simulink model "regulator_ver2"  (Simulink 8.4)
settings: Solver=ode5  StartTime=0.0  StopTime=500  FixedStep=0.05  RelTol=1e-3
values from neighbouring files (symbols this model uses):
  a = 31    [charakterystyka_pompa.m]    (also in charakterystyka_pompa_sterownik.m; dane14listopad.mat; danePompa.mat; pomiary.m)
  b = 40    [charakterystyki_zawory_reczne.m]    (also in daneZawory_cz2.mat; pomiary.m; rhs.m)
  c = p(1)    [cel.m]    (also in charakterystyki_zawory_reczne.m = 10; daneZawory_cz2.mat = 10; identyfikacja_parametrow.m = 10; identyfikacja_zawor2.m = 10)
  C1 = q/sqrt(H1pp)    [linearyzacja_analitycznie.m]    (also in wskaznikZawor1.m = parametry(1))
  C2 = q/sqrt(H2pp)    [linearyzacja_analitycznie.m]    (also in wskaznikZawor2.m = parametry(1))
  C3 = q/sqrt(H3pp)    [linearyzacja_analitycznie.m]    (also in wskaznikZawor3.m = parametry(1))
  H2max = 40    [charakterystyki_zawory_reczne.m]    (also in daneZawory_cz2.mat; pomiary.m)
  R = 40    [charakterystyki_zawory_reczne.m]    (also in daneZawory_cz2.mat; nastawyLQ.m; pomiary.m; rhs.m)
  w = 5    [charakterystyka_pompa.m]    (also in charakterystyka_pompa_sterownik.m; dane14listopad.mat; danePompa.mat; pomiary.m)
settings Model: Creator=Michal  LastModifiedBy=Michal
settings DataIOCC: SignalLoggingSaveFormat=Dataset
settings OptimizationCC: ExpressionDepthLimit=128
settings DebuggingCC: ArtificialAlgebraicLoopMsg=none  FcnCallInpInsideContextMsg=EnableAllAsError  StateNameClashWarn=none
settings GRTTargetCC: CombineOutputUpdateFcns=on  GRTInterface=off
settings ConfigComp: Description=PLC Coder Custom Configuration Component  PLC_TargetIDE=pcworx60  PLC_GenerateReport=off

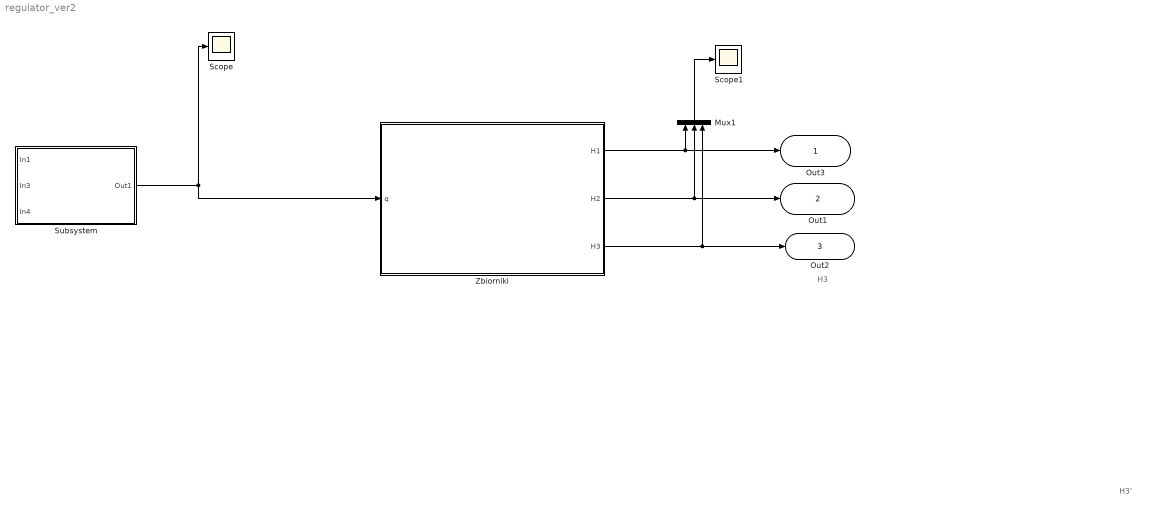
== system regulator_ver2 ==
  note: H3
  note: H3'
  Mux1 : Mux  Inputs=3
  Scope : Scope
      settings: TimeRange=500  SaveName=q_lqr
  Scope1 : Scope
      settings: TimeRange=500  YMin=-300000  YMax=50000  SaveName=H_lqr
  Subsystem : Subsystem  TreatAsAtomicUnit=on
      settings: MinAlgLoopOccurrences=on
  Zbiorniki : Subsystem
  Out3 : Outport
  Out1 : Outport  Port=2
  Out2 : Outport  Port=3
  wires:
  Zbiorniki/3(H3) -> Out2/1, Mux1/3
  Zbiorniki/1(H1) -> Mux1/1, Out3/1
  Zbiorniki/2(H2) -> Mux1/2, Out1/1
  Mux1/1 -> Scope1/1
  Subsystem/1(Out1) -> Zbiorniki/1(q), Scope/1

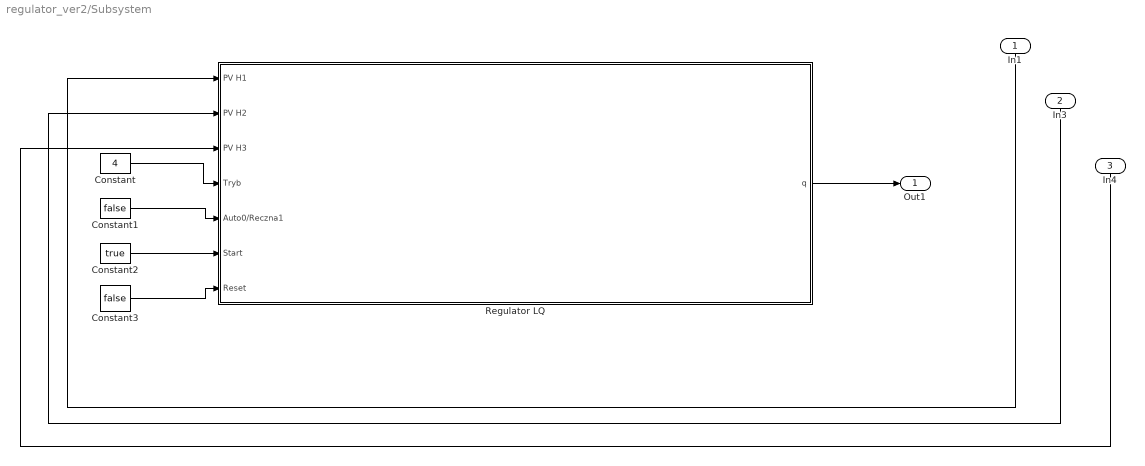
== system regulator_ver2/Subsystem ==
  In1 : Inport  OutDataTypeStr=single
  In3 : Inport  Port=2  OutDataTypeStr=single
  In4 : Inport  Port=3  OutDataTypeStr=single
  Constant : Constant  Value=4  OutDataTypeStr=uint16
  Constant1 : Constant  Value=false  OutMin=0  OutMax=1  OutDataTypeStr=boolean
  Constant2 : Constant  Value=true  OutMin=0  OutMax=1  OutDataTypeStr=boolean
  Constant3 : Constant  Value=false  OutMin=0  OutMax=1  OutDataTypeStr=boolean
  Regulator LQ : Subsystem  TreatAsAtomicUnit=on
      settings: MinAlgLoopOccurrences=on
  Out1 : Outport
  wires:
  In1/1 -> Regulator LQ/1(PV H1)
  In4/1 -> Regulator LQ/3(PV H3)
  In3/1 -> Regulator LQ/2(PV H2)
  Constant/1 -> Regulator LQ/4(Tryb)
  Constant1/1 -> Regulator LQ/5(Auto0/Reczna1)
  Regulator LQ/1(q) -> Out1/1
  Constant2/1 -> Regulator LQ/6(Start)
  Constant3/1 -> Regulator LQ/7(Reset)

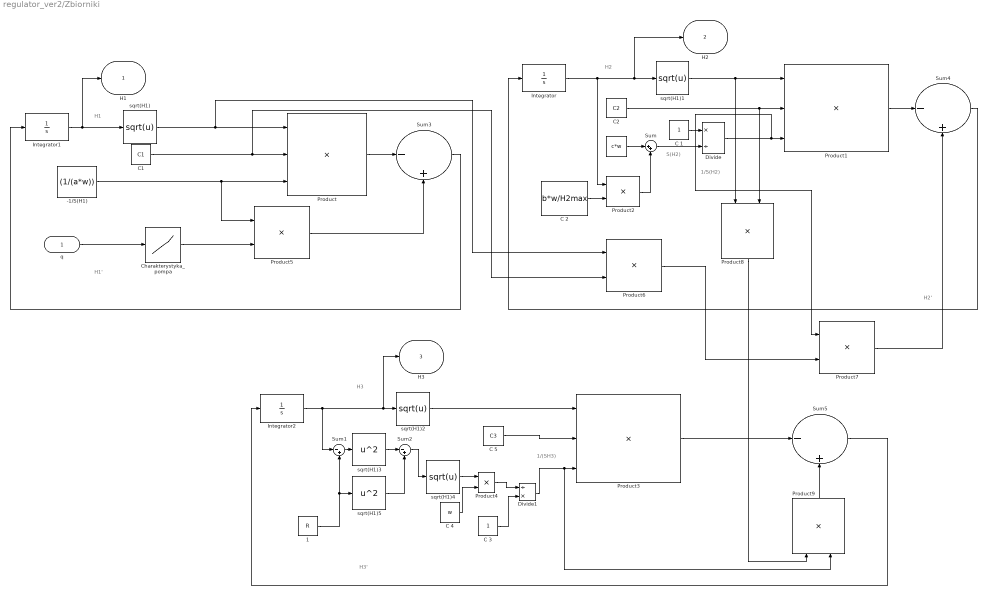
== system regulator_ver2/Zbiorniki ==
  note: H1
  note: 1/S(H2)
  note: S(H2)
  note: H2'
  note: H2
  note: 1/(SH3)
  note: H3
  note: H1'
  note: H3'
  q : Inport
  " " : Constant  Value=c*w
  " 1" : Constant  Value=R
  -1/S(H1) : Constant  Value=(1/(a*w))
  C 1 : Constant
  C 2 : Constant  Value=b*w/H2max
  C 3 : Constant
  C 4 : Constant  Value=w
  C 5 : Constant  Value=C3
  "C1 " : Constant  Value=C1
  "C2 " : Constant  Value=C2
  Charakterystyka_pompa : Lookup_n-D  NumberOfTableDimensions=1  BreakpointsForDimension1="[0.300000000000000\t0.305000000000000\t0.310000000000000\t0.315000000000000\t0.320000000000000\t0.325000000000000\t0.330000000000000\t0.335000000000000\t0.340000000000000\t0.345000000000000\t0.350000000000000\t0.355000000000000\t0.360000000000000\t0.365000000000000\t0.370000000000000\t0.375000000000000\t0.380000000000000\t0.385000000000000\t0.390000000000000\t0.395000000000000\t0.400000000000000\t0.405000000000000\t0.410000000000000\t0.415000000000000\t0.420000000000000\t0.425000000000000\t0.430000000000000\t0.435000000000000\t0.440000000000000\t0.445000000000000\t0.450000000000000\t0.455000000000000\t0.460000000000000\t0.465000000000000\t0.470000000000000\t0.475000000000000\t0.480000000000000\t0.485000000000000\t0.490000000000000\t0.495000000000000\t0.500000000000000\t0.505000000000000\t0.510000000000000\t0.515000000000000\t0.520000000000000\t0.525000000000000\t0.530000000000000\t0.535000000000000\t0.540000000000000\t0.545000000000000\t0.550000000000000\t0.555000000000000\t0.560000000000000\t0.565000000000000\t0.570000000000000\t0.575000000000000\t0.580000000000000\t0.585000000000000\t0.590000000000000\t0.595000000000000\t0.600000000000000\t0.605000000000000\t0.610000000000000\t0.615000000000000\t0.620000000000000\t0.625000000000000\t0.630000000000000\t0.635000000000000\t0.640000000000000\t0.645000000000000\t0.650000000000000\t0.655000000000000\t0.660000000000000\t0.665000000000000\t0.670000000000000\t0.675000000000000\t0.680000000000000\t0.685000000000000\t0.690000000000000\t0.695000000000000\t0.700000000000000\t0.705000000000000\t0.710000000000000\t0.715000000000000\t0.720000000000000\t0.725000000000000\t0.730000000000000\t0.735000000000000\t0.740000000000000\t0.745000000000000\t0.750000000000000\t0.755000000000000\t0.760000000000000\t0.765000000000000\t0.770000000000000\t0.775000000000000\t0.780000000000000\t0.785000000000000\t0.790000000000000\t0.795000000000000\t0.800000000000000\t0.805000000000000\t0.810000000000000\t0.815000000000000\t0.820000000000000\t0.825000000000000\t0.830000000000000\t0.835000000000000\t0.840000000000000\t0.845000000000000\t0.850000000000000\t0.855000000000000\t0.860000000000000\t0.865000000000000\t0.870000000000000\t0.875000000000000\t0.880000000000000\t0.885000000000000\t0.890000000000000\t0.895000000000000\t0.900000000000000\t0.905000000000000\t0.910000000000000\t0.915000000000000\t0.920000000000000\t0.925000000000000\t0.930000000000000\t0.935000000000000\t0.940000000000000\t0.945000000000000\t0.950000000000000\t0.955000000000000\t0.960000000000000\t0.965000000000000\t0.970000000000000\t0.975000000000000\t0.980000000000000\t0.985000000000000\t0.990000000000000\t0.995000000000000\t1]"  Table="[10.4471978396270\t11.7296031510510\t13.0028115267443\t14.2669102745871\t15.5219867024602\t16.7681281182441\t18.0054218298192\t19.2339551450661\t20.4538153718654\t21.6650898180975\t22.8678657916430\t24.0622306003825\t25.2482715521964\t26.4260759549652\t27.5957311165696\t28.7573243448901\t29.9109429478071\t31.0566742332013\t32.1946055089531\t33.3248240829430\t34.4474172630516\t35.5624723571595\t36.6700766731472\t37.7703175188951\t38.8632822022838\t39.9490580311939\t41.0277323135059\t42.0993923571003\t43.1641254698577\t44.2220189596585\t45.2731601343833\t46.3176363019127\t47.3555347701271\t48.3869428469072\t49.4119478401333\t50.4306370576861\t51.4430978074461\t52.4494173972938\t53.4496831351098\t54.4439823287746\t55.4324022861686\t56.4150303151725\t57.3919537236668\t58.3632598195320\t59.3290359106486\t60.2893693048972\t61.2443473101582\t62.1940572343123\t63.1385863852399\t64.0780220708216\t65.0124515989380\t65.9419622774695\t66.8666414142967\t67.7865763173000\t68.7018542943601\t69.6125626533575\t70.5187887021727\t71.4206197486861\t72.3181431007785\t73.2114460663303\t74.1006159532220\t74.9857400693341\t75.8669057225472\t76.7442002207418\t77.6177108717985\t78.4875249835977\t79.3537298640200\t80.2164128209460\t81.0756611622562\t81.9315621958310\t82.7842032295510\t83.6336715712968\t84.4800545289489\t85.3234394103878\t86.1639135234941\t87.0015641761482\t87.8364786762308\t88.6687443316223\t89.4984484502032\t90.3256783398542\t91.1505213084557\t91.9730646638883\t92.7933957140324\t93.6116017667686\t94.4277701299776\t95.2419881115397\t96.0543430193355\t96.8649221612455\t97.6738128451504\t98.4811023789305\t99.2868780704665\t100.091227227639\t100.894237158328\t101.695995170415\t102.496588571779\t103.296104670302\t104.094630773865\t104.892254190346\t105.689062227628\t106.485142193590\t107.280581396114\t108.075467143079\t108.869886742366\t109.663927501857\t110.457676729430\t111.251221732967\t112.044649820349\t112.838048299455\t113.631504478167\t114.425105664364\t115.218939165928\t116.013092290739\t116.807652346678\t117.602706641625\t118.398342483460\t119.194647180064\t119.991708039318\t120.789612369102\t121.588447477297\t122.388300671783\t123.189259260441\t123.991410551151\t124.794841851793\t125.599640470250\t126.405893714400\t127.213688892124\t128.023113311303\t128.834254279818\t129.647199105549\t130.462035096376\t131.278849560181\t132.097729804843\t132.918763138243\t133.742036868262\t134.567638302780\t135.395654749677\t136.226173516835\t137.059281912134\t137.895067243454\t138.733616818676\t139.575017945680]"  InternalRulePriority=Speed  RndMeth=Simplest  InputSameDT=on
  Divide : Product  Inputs=*/
  Divide1 : Product  Inputs=/*
  Integrator : Integrator  InitialCondition=0.01
  Integrator1 : Integrator  InitialCondition=0.01
  Integrator2 : Integrator  InitialCondition=0.01
  Product : Product  Inputs=3
  Product1 : Product  Inputs=3
  Product{2,4..9} (7 alike) : Product
  Product3 : Product  Inputs=3
  Sum : Sum  Inputs=|++
  Sum{1..5} (5 alike) : Sum  Inputs=|-+
  sqrt(H1){,1..2,4} (4 alike) : Fcn  Expr=sqrt(u)
  sqrt(H1)3 : Fcn  Expr=u^2
  sqrt(H1)5 : Fcn  Expr=u^2
  H1 : Outport
  H2 : Outport  Port=2
  H3 : Outport  Port=3
  wires:
  Product1/1 -> Sum4/1
  Product/1 -> Sum3/1
  Product5/1 -> Sum3/2
  Sum4/1 -> Integrator/1
  Sum5/1 -> Integrator2/1
  Sum3/1 -> Integrator1/1
  Product7/1 -> Sum4/2
  Product6/1 -> Product7/2
  Integrator/1 -> Product2/1, H2/1, sqrt(H1)1/1
  Product9/1 -> Sum5/2
  sqrt(H1)/1 -> Product6/1, Product/1
  Integrator1/1 -> H1/1, sqrt(H1)/1
  -1/S(H1)/1 -> Product5/1, Product/3
  "C1 "/1 -> Product6/2, Product/2
  sqrt(H1)5/1 -> Sum2/2
  Divide1/1 -> Product9/2, Product3/3
  C 4/1 -> Product4/2
  Product4/1 -> Divide1/1
  C 3/1 -> Divide1/2
  C 5/1 -> Product3/2
  sqrt(H1)2/1 -> Product3/1
  " 1"/1 -> sqrt(H1)5/1, Sum1/2
  Sum2/1 -> sqrt(H1)4/1
  Sum1/1 -> sqrt(H1)3/1
  sqrt(H1)4/1 -> Product4/1
  sqrt(H1)3/1 -> Sum2/1
  Integrator2/1 -> H3/1, sqrt(H1)2/1, Sum1/1
  Product3/1 -> Sum5/1
  Divide/1 -> Product1/3, Product7/1
  C 1/1 -> Divide/1
  Sum/1 -> Divide/2
  Product2/1 -> Sum/2
  C 2/1 -> Product2/2
  " "/1 -> Sum/1
  "C2 "/1 -> Product1/2, Product8/2
  sqrt(H1)1/1 -> Product1/1, Product8/1
  Product8/1 -> Product9/1
  Charakterystyka_pompa/1 -> Product5/2
  q/1 -> Charakterystyka_pompa/1

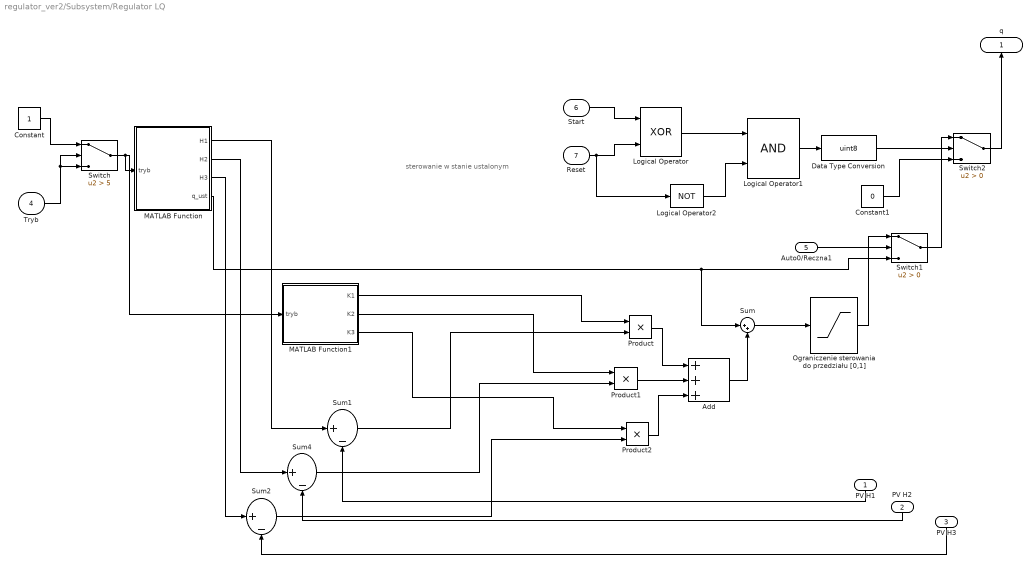
== system regulator_ver2/Subsystem/Regulator LQ ==
  note: sterowanie w stanie ustalonym
  PV H1 : Inport  OutDataTypeStr=single
  PV H2 : Inport  Port=2  OutDataTypeStr=single
  PV H3 : Inport  Port=3  OutDataTypeStr=single
  Tryb : Inport  Port=4  OutDataTypeStr=uint16
  Auto0/Reczna1 : Inport  Port=5  OutMin=0  OutMax=1  OutDataTypeStr=boolean
  Start : Inport  Port=6  OutDataTypeStr=boolean
  Reset : Inport  Port=7  OutDataTypeStr=boolean
  Add : Sum  Inputs=+++  AccumDataTypeStr=single
  Constant : Constant  OutDataTypeStr=uint16
  Constant1 : Constant  Value=0  OutDataTypeStr=single
  Data Type Conversion : DataTypeConversion  OutDataTypeStr=uint8
  Logical Operator : Logic  Operator=XOR  AllPortsSameDT=off  OutDataTypeStr=boolean
  Logical Operator1 : Logic  AllPortsSameDT=off  OutDataTypeStr=boolean
  Logical Operator2 : Logic  Operator=NOT  AllPortsSameDT=off  OutDataTypeStr=boolean
  MATLAB Function : MATLAB Function  TreatAsAtomicUnit=on
  MATLAB Function1 : MATLAB Function  TreatAsAtomicUnit=on
  Ograniczenie sterowania do przedziału [0,1] : Saturate  UpperLimit=1  LowerLimit=0  OutDataTypeStr=single
  Product : Product
  Product1 : Product
  Product2 : Product
  Sum : Sum  Inputs=|++  OutDataTypeStr=single
  Sum1 : Sum  Inputs=|+-  AccumDataTypeStr=single  OutDataTypeStr=single
  Sum2 : Sum  Inputs=|+-  OutDataTypeStr=single
  Sum4 : Sum  Inputs=|+-  OutDataTypeStr=single
  Switch : Switch  Criteria=u2 > Threshold  Threshold=5  OutDataTypeStr=uint16
  Switch1 : Switch  Criteria=u2 > Threshold  OutMin=0  OutMax=1  OutDataTypeStr=single
  Switch2 : Switch  Criteria=u2 > Threshold  OutMin=0  OutMax=1  OutDataTypeStr=single
  q : Outport
  wires:
  PV H1/1 -> Sum1/2
  PV H3/1 -> Sum2/2
  PV H2/1 -> Sum4/2
  Switch/1 -> MATLAB Function1/1(tryb), MATLAB Function/1(tryb)
  Sum1/1 -> Product/2
  Sum4/1 -> Product1/2
  Sum2/1 -> Product2/2
  Product/1 -> Add/1
  Product1/1 -> Add/2
  Product2/1 -> Add/3
  Add/1 -> Sum/2
  Sum/1 -> Ograniczenie sterowania do przedziału [0,1]/1
  Tryb/1 -> Switch/2, Switch/3
  Constant/1 -> Switch/1
  Auto0/Reczna1/1 -> Switch1/2
  Start/1 -> Logical Operator/1
  Reset/1 -> Logical Operator2/1, Logical Operator/2
  Logical Operator/1 -> Logical Operator1/1
  Logical Operator2/1 -> Logical Operator1/2
  Logical Operator1/1 -> Data Type Conversion/1
  Data Type Conversion/1 -> Switch2/2
  Switch2/1 -> q/1
  Constant1/1 -> Switch2/3
  Ograniczenie sterowania do przedziału [0,1]/1 -> Switch1/1
  Switch1/1 -> Switch2/1
  MATLAB Function/1(H1) -> Sum1/1
  MATLAB Function/2(H2) -> Sum4/1
  MATLAB Function/3(H3) -> Sum2/1
  MATLAB Function/4(q_ust) -> Switch1/3, Sum/1
  MATLAB Function1/3(K3) -> Product2/1
  MATLAB Function1/2(K2) -> Product1/1
  MATLAB Function1/1(K1) -> Product/1

== matlab function Subsystem/Regulator LQ/MATLAB Function1 ==
  data: tryb input double; K1 output double; K2 output double; K3 output double
function [K1,K2,K3]=Wzmocnienie(tryb)
    P=[0.0314 0.0142 0.01;0.0355 0.0168 0.0106; 0.0349 0.0188 0.0108; 0.0376 0.0227 0.0122; 0.0834 0.0440 0.0108];
    K1=P(tryb,1);
    K2=P(tryb,2);
    K3=P(tryb,3);
end

== matlab function Subsystem/Regulator LQ/MATLAB Function ==
  data: H1 output double; tryb input double; H2 output double; H3 output double; q_ust output double
function [H1,H2,H3,q_ust]  = Punkty_pracy(tryb)
    Poziom1=[5.5 7.7 10 12.6 10.3];
    Poziom2=[9.8 13.7 17.4 22.1 23.5];
    Poziom3=[7.8 10 12 15 11.4];
    sterowanie=[0.6 0.65 0.7 0.75 0.8];
    H1=Poziom1(tryb);
    H2=Poziom2(tryb);
    H3=Poziom3(tryb);
    q_ust=sterowanie(tryb);
    
end
